simulink model "FSK_Hamming"  (R2018b)
settings: Solver=VariableStepAuto  StartTime=0.0  StopTime=10.0  RelTol=1e-3
values from neighbouring files (symbols this model uses):
  BitRate = 10000    [FSK.m]
  MessageLength = 26    [FSK.m]
  x = -10:1:20    [FSK.m]    (also in compare.m = -10:1:15)
undefined symbols (not defined in the file or in its folder): i
libraries: commblkcod2 x2, commdigbbndfm2 x2, commchan3 x1, commsink2 x1, commrandsrc3 x1
settings Model: Creator=Aurora  LastModifiedBy=Aurora

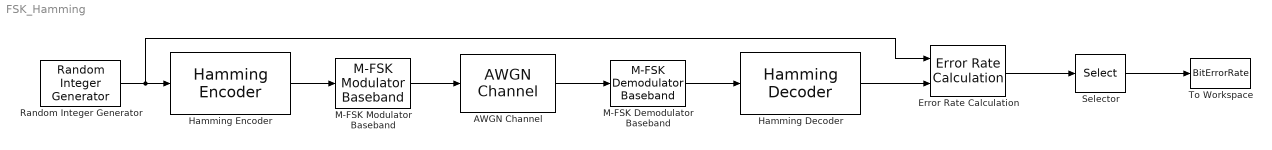
== system FSK_Hamming ==
  AWGN Channel : commchan3/AWGN Channel  InputProcessing=Columns as channels (frame based)  seed=67  noiseMode="Signal to noise ratio  (SNR)"  EbNodB=10  EsNodB=10  SNRdB=x(i)  bitsPerSym=1  Ps=1  Tsym=1  variance=1
  Error Rate Calculation : commsink2/Error Rate Calculation  N=0  st_delay=0  cp_mode=Entire frame  subframe=[]  PMode=Port  WsName=ErrorVec  RsMode2=off  stop=off  numErr=100  maxBits=1e6
  Hamming Decoder : commblkcod2/Hamming Decoder  n=CodewordLength  k=MessageLength
      settings: SourceProductName=Communications System Toolbox  SourceProductBaseCode=CM
  Hamming Encoder : commblkcod2/Hamming Encoder  n=CodewordLength  k=MessageLength
      settings: SourceProductName=Communications System Toolbox  SourceProductBaseCode=CM
  M-FSK Demodulator Baseband : commdigbbndfm2/M-FSK Demodulator Baseband  M=2  OutType=Bit  Dec=Binary  freqSep=1000  numSamp=17  RateOptions=Enforce single-rate processing  outDataType=double
      settings: SourceProductName=Communications System Toolbox  SourceProductBaseCode=CM
  M-FSK Modulator Baseband : commdigbbndfm2/M-FSK Modulator Baseband  M=2  InType=Bit  Enc=Binary  freqSep=2000  phaseType=Continuous  numSamp=17  RateOptions=Enforce single-rate processing  outDataType=double
      settings: SourceProductName=Communications System Toolbox
  Random Integer Generator : commrandsrc3/Random Integer Generator  SetSize=2  SeedSource=Parameter  Seed=37  SampleTime=1/BitRate  SamplesPerFrame=MessageLength  OutputDataType=double  SimulateUsing=Interpreted execution
  Selector : Selector  InputPortWidth=3  IndexOptions=Index vector (dialog)  Indices=[1]  OutputSizes=1
  To Workspace : ToWorkspace  VariableName=BitErrorRate  SampleTime=-1
  wires:
  Hamming Decoder/1 -> Error Rate Calculation/2
  M-FSK Modulator Baseband/1 -> AWGN Channel/1
  Hamming Encoder/1 -> M-FSK Modulator Baseband/1
  Error Rate Calculation/1 -> Selector/1
  M-FSK Demodulator Baseband/1 -> Hamming Decoder/1
  Random Integer Generator/1 -> Error Rate Calculation/1, Hamming Encoder/1
  Selector/1 -> To Workspace/1
  AWGN Channel/1 -> M-FSK Demodulator Baseband/1
